simulink model "LATC_Test_Calc"  (R2021b)
settings: Solver=FixedStepDiscrete  StartTime=3849.7586  StopTime=3889.7825  FixedStep=0.01  RelTol=1e-3
values from neighbouring files (symbols this model uses):
  P_Global_CharSpd_ms : value not decoded    [PubParsGlobal.sldd]
  P_Global_SteeringAngleRatio : value not decoded    [PubParsGlobal.sldd]
  P_Global_WheelBase_m : value not decoded    [PubParsGlobal.sldd]
  P_LCS_CycleTime = 0.4 0.4 0.4 0.4 0.4 0.4 0.4 0.4 0.4 0.6 0.6 0.6 0.6 0.6 0.6 0.6 0.4 0.4 0.4 0.4 0.4 0.4 0.4 0.4 0.4 0.6 0.6 0.6 0.6 0.6 0.6 0.6 0.4 0.4 0.4 0.4 0.4 0.4 0.4 0.4 0.4 0.6 0.6 0.6 0.6 0.6 0.6 0.6 0.4 0.4 0.4 0.4 0.4 0.4 0.4 0.4 0.4 0.6 0.6 0.6 0.6 0.6 0.6 0.6 0.4 0.4 0.4 0.4 0.4 0.4 0.4 0.4 0.4 0.6 0.6 0.6 0.6 0.6 0.6 0.6 0.4 0.4 0.4 0.4 0.4 0.4 0.4 0.4 0.4 0.6 0.6 0.6 0.6 0.6 0.6 0.6 0.4 0.4 0.4 0.4    [LATC.sldd]
  P_LCS_ESS_AngleSlope_Limit = 2.9    [LATC.sldd]    (also in LCS_v05.sldd)
  P_LCS_LATC_CurOffsetVehicleSpdLimitValue_degs = 7.0    [LATC.sldd]
  P_LCS_LATC_ELKAngleSlope_ratio : value not decoded    [LATC.sldd]
  P_LCS_LATC_ELKMaxLatAcc_ms2 : value not decoded    [LATC.sldd]
  P_LCS_LATC_ESSAngleSlope_ratio : value not decoded    [LATC.sldd]
  P_LCS_LATC_ESSMaxLatAcc_ms2 : value not decoded    [LATC.sldd]
  P_LCS_LATC_LCAngleSlope_ratio : value not decoded    [LATC.sldd]
  P_LCS_LATC_LCCancleMaxLatAcc_ms2 : value not decoded    [LATC.sldd]
  P_LCS_LATC_LCEcoAngleSlope_ratio : value not decoded    [LATC.sldd]
  P_LCS_LATC_LCEcoMaxLatAcc_ms2 : value not decoded    [LATC.sldd]
  P_LCS_LATC_LCKAngleSlope_ratio : value not decoded    [LATC.sldd]
  P_LCS_LATC_LCKIEAngleSlope_ratio : value not decoded    [LATC.sldd]
  P_LCS_LATC_LCKIEMaxLatAcc_ms2 : value not decoded    [LATC.sldd]
  P_LCS_LATC_LCKMaxLatAcc_ms2 : value not decoded    [LATC.sldd]
  P_LCS_LATC_LCNormalAngleSlope_ratio : value not decoded    [LATC.sldd]
  P_LCS_LATC_LCNormalMaxLatAcc_ms2 : value not decoded    [LATC.sldd]
  P_LCS_LATC_LCSportAngleSlope_ratio : value not decoded    [LATC.sldd]
  P_LCS_LATC_LCSportMaxLatAcc_ms2 : value not decoded    [LATC.sldd]
  P_LCS_LATC_LKAAngleSlope_ratio : value not decoded    [LATC.sldd]
  P_LCS_LATC_LKAMaxLatAcc_ms2 : value not decoded    [LATC.sldd]
  P_LCS_LATC_MatrixQ1_st = 0.8 0.8 1.2 1.4 1.4 1.4 2.0 2.2 2.2 2.2 2.2 2.2 2.2 2.2 2.2 2.2 0.8 0.8 1.2 1.4 1.4 1.4 2.0 2.2 2.2 2.2 2.2 2.2 2.2 2.2 2.2 2.2 0.8 0.8 1.2 1.4 1.4 1.4 2.0 2.2 2.2 2.2 2.2 2.2 2.2 2.2 2.2 2.2 0.8 0.8 1.2 1.4 1.4 1.4 2.0 2.2 2.2 2.2 2.2 2.2 2.2 2.2 2.2 2.2 0.8 0.8 1.2 1.4 1.4 1.4 2.0 2.2 2.2 2.2 2.2 2.2 2.2 2.2 2.2 2.2 0.8 0.8 1.2 1.4 1.4 1.4 2.0 2.2 2.2 2.2 2.2 2.2 2.2 2.2 2.2 2.2 0.8 0.8 1.2 1.4    [LATC.sldd]
  P_LCS_LATC_MatrixQ3_st = 20.0 20.0 20.0 20.0 20.0 15.0 15.0 15.0 15.0 15.0 15.0 15.0 15.0 13.0 13.0 13.0 20.0 20.0 20.0 20.0 20.0 15.0 15.0 15.0 15.0 15.0 15.0 15.0 15.0 13.0 13.0 13.0 20.0 20.0 20.0 20.0 20.0 15.0 15.0 15.0 15.0 15.0 15.0 15.0 15.0 13.0 13.0 13.0 20.0 20.0 20.0 20.0 20.0 15.0 15.0 15.0 15.0 15.0 15.0 15.0 15.0 13.0 13.0 13.0 20.0 20.0 20.0 20.0 20.0 15.0 15.0 15.0 15.0 15.0 15.0 15.0 15.0 13.0 13.0 13.0    [LATC.sldd]
  P_LCS_LATC_MatrixR_st = 10.0 10.0 10.0 10.0 10.0 10.0 10.0 15.0 15.0 15.0 15.0 15.0 15.0 15.0 15.0 15.0 10.0 10.0 10.0 10.0 10.0 10.0 10.0 15.0 15.0 15.0 15.0 15.0 15.0 15.0 15.0 15.0 10.0 10.0 10.0 10.0 10.0 10.0 10.0 15.0 15.0 15.0 15.0 15.0 15.0 15.0 15.0 15.0 10.0 10.0 10.0 10.0 10.0 10.0 10.0 15.0 15.0 15.0 15.0 15.0 15.0 15.0 15.0 15.0 10.0 10.0 10.0 10.0 10.0 10.0 10.0 15.0 15.0 15.0 15.0 15.0 15.0 15.0 15.0 15.0    [LATC.sldd]
  P_LCS_LATC_StateActivAngleSlopeLimit_ratio : value not decoded    [LATC.sldd]
  P_LCS_LATC_StateActiveFlg_TabX_st : value not decoded    [LATC.sldd]
  P_LCS_LATC_StateActiveHoldTime_TabY_st : value not decoded    [LATC.sldd]
  P_LCS_LATC_StateHoldTime_st = 250.0    [LATC.sldd]
  P_LCS_LATC_TarAngleFliterWindowSize = 5.0    [LATC.sldd]
  P_LCS_LineVaildSW = 0.0    [LATC.sldd]
  P_LCS_Lookahead_Distance : value not decoded    [LATC.sldd]
  P_LCS_VehicleSpd_TabX_Kph : value not decoded    [LATC.sldd]
libraries: simulink x4
(part 3 of 4)

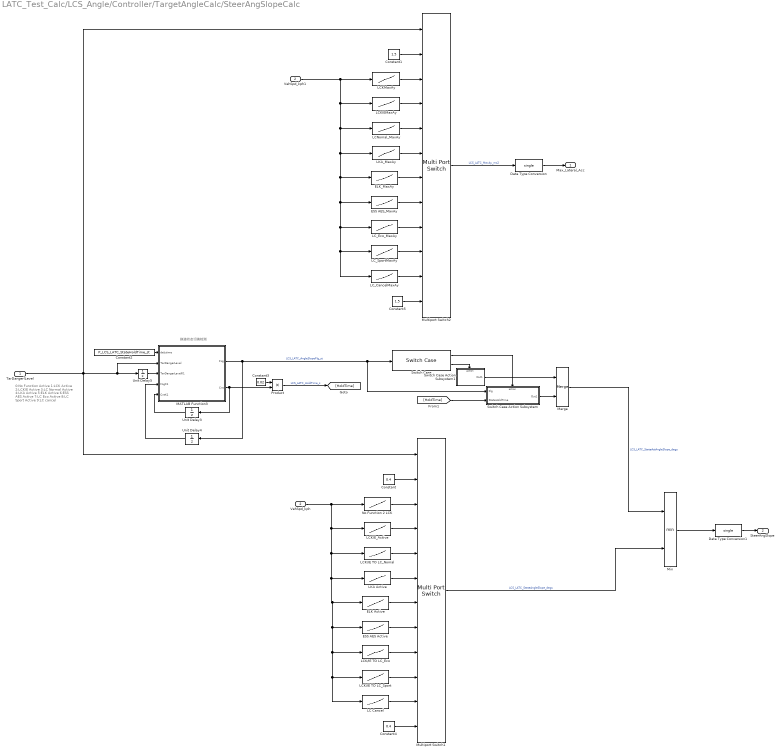
== system LATC_Test_Calc/LCS_Angle/Controller/TargetAngleCalc/SteerAngSlopeCalc ==
  note: 换道状态切换检测
  note: 0:No Function Active
      | 1:LCK Active
      | 2:LCKIE Active
      | 3:LC Normal Active
      | 4:LKA Active
      | 5:ELK Active
      | 6:ESS AES Active
      | 7:LC Eco Active
      | 8:LC Sport Active
      | 9:LC cancel
  TarDangerlLevel : Inport
  VehSpd_kph : Inport  Port=2
  Constant : Constant  Value=0.4  OutDataTypeStr=single
  Constant1 : Constant  Value=1.5  OutDataTypeStr=single
  Constant2 : Constant  Value=P_LCS_LATC_StateHoldTime_st  OutDataTypeStr=uint16
  Constant3 : Constant  Value=0.02
  Constant4 : Constant  Value=0.4  OutDataTypeStr=single
  Constant5 : Constant  Value=1.5  OutDataTypeStr=single
  Data Type Conversion : DataTypeConversion  OutDataTypeStr=single
  Data Type Conversion1 : DataTypeConversion  OutDataTypeStr=single
  ELK Active : Lookup_n-D  NumberOfTableDimensions=1  BreakpointsForDimension1=P_LCS_VehicleSpd_TabX_Kph  Table=P_LCS_LATC_ELKAngleSlope_ratio  ExtrapMethod=Clip  InternalRulePriority=Speed  RndMeth=Simplest  InputSameDT=on
  ELK_MaxAy : Lookup_n-D  NumberOfTableDimensions=1  BreakpointsForDimension1=P_LCS_VehicleSpd_TabX_Kph  Table=P_LCS_LATC_ELKMaxLatAcc_ms2  ExtrapMethod=Clip  InternalRulePriority=Speed  RndMeth=Simplest  InputSameDT=on
  ESS AES Active : Lookup_n-D  NumberOfTableDimensions=1  BreakpointsForDimension1=P_LCS_VehicleSpd_TabX_Kph  Table=P_LCS_LATC_ESSAngleSlope_ratio  ExtrapMethod=Clip  InternalRulePriority=Speed  RndMeth=Simplest  InputSameDT=on
  ESS AES_MaxAy : Lookup_n-D  NumberOfTableDimensions=1  BreakpointsForDimension1=P_LCS_VehicleSpd_TabX_Kph  Table=P_LCS_LATC_ESSMaxLatAcc_ms2  ExtrapMethod=Clip  InternalRulePriority=Speed  RndMeth=Simplest  InputSameDT=on
  LC Cancel : Lookup_n-D  NumberOfTableDimensions=1  BreakpointsForDimension1=P_LCS_VehicleSpd_TabX_Kph  Table=P_LCS_LATC_LCAngleSlope_ratio  ExtrapMethod=Clip  InternalRulePriority=Speed  RndMeth=Simplest  InputSameDT=on
  LCK/IE TO LC_Eco : Lookup_n-D  NumberOfTableDimensions=1  BreakpointsForDimension1=P_LCS_VehicleSpd_TabX_Kph  Table=P_LCS_LATC_LCEcoAngleSlope_ratio  ExtrapMethod=Clip  InternalRulePriority=Speed  RndMeth=Simplest  InputSameDT=on
  LCK/IE TO LC_Nomal : Lookup_n-D  NumberOfTableDimensions=1  BreakpointsForDimension1=P_LCS_VehicleSpd_TabX_Kph  Table=P_LCS_LATC_LCNormalAngleSlope_ratio  ExtrapMethod=Clip  InternalRulePriority=Speed  RndMeth=Simplest  InputSameDT=on
  LCK/IE TO LC_Sport : Lookup_n-D  NumberOfTableDimensions=1  BreakpointsForDimension1=P_LCS_VehicleSpd_TabX_Kph  Table=P_LCS_LATC_LCSportAngleSlope_ratio  ExtrapMethod=Clip  InternalRulePriority=Speed  RndMeth=Simplest  InputSameDT=on
  LCKIEMaxAy : Lookup_n-D  NumberOfTableDimensions=1  BreakpointsForDimension1=P_LCS_VehicleSpd_TabX_Kph  Table=P_LCS_LATC_LCKIEMaxLatAcc_ms2  ExtrapMethod=Clip  InternalRulePriority=Speed  RndMeth=Simplest  InputSameDT=on
  LCKIE_Active : Lookup_n-D  NumberOfTableDimensions=1  BreakpointsForDimension1=P_LCS_VehicleSpd_TabX_Kph  Table=P_LCS_LATC_LCKIEAngleSlope_ratio  ExtrapMethod=Clip  InternalRulePriority=Speed  RndMeth=Simplest  InputSameDT=on
  LCKMaxAy : Lookup_n-D  NumberOfTableDimensions=1  BreakpointsForDimension1=P_LCS_VehicleSpd_TabX_Kph  Table=P_LCS_LATC_LCKMaxLatAcc_ms2  ExtrapMethod=Clip  InternalRulePriority=Speed  RndMeth=Simplest  InputSameDT=on
  LCNomal_MaxAy : Lookup_n-D  NumberOfTableDimensions=1  BreakpointsForDimension1=P_LCS_VehicleSpd_TabX_Kph  Table=P_LCS_LATC_LCNormalMaxLatAcc_ms2  ExtrapMethod=Clip  InternalRulePriority=Speed  RndMeth=Simplest  InputSameDT=on
  LC_CancelMaxAy : Lookup_n-D  NumberOfTableDimensions=1  BreakpointsForDimension1=P_LCS_VehicleSpd_TabX_Kph  Table=P_LCS_LATC_LCCancleMaxLatAcc_ms2  ExtrapMethod=Clip  InternalRulePriority=Speed  RndMeth=Simplest  InputSameDT=on
  LC_Eco_MaxAy : Lookup_n-D  NumberOfTableDimensions=1  BreakpointsForDimension1=P_LCS_VehicleSpd_TabX_Kph  Table=P_LCS_LATC_LCEcoMaxLatAcc_ms2  ExtrapMethod=Clip  InternalRulePriority=Speed  RndMeth=Simplest  InputSameDT=on
  LC_SportMaxAy : Lookup_n-D  NumberOfTableDimensions=1  BreakpointsForDimension1=P_LCS_VehicleSpd_TabX_Kph  Table=P_LCS_LATC_LCSportMaxLatAcc_ms2  ExtrapMethod=Clip  InternalRulePriority=Speed  RndMeth=Simplest  InputSameDT=on
  LKA Active : Lookup_n-D  NumberOfTableDimensions=1  BreakpointsForDimension1=P_LCS_VehicleSpd_TabX_Kph  Table=P_LCS_LATC_LKAAngleSlope_ratio  ExtrapMethod=Clip  InternalRulePriority=Speed  RndMeth=Simplest  InputSameDT=on
  LKA_MaxAy : Lookup_n-D  NumberOfTableDimensions=1  BreakpointsForDimension1=P_LCS_VehicleSpd_TabX_Kph  Table=P_LCS_LATC_LKAMaxLatAcc_ms2  ExtrapMethod=Clip  InternalRulePriority=Speed  RndMeth=Simplest  InputSameDT=on
  MATLAB Function3 : MATLAB Function  TreatAsAtomicUnit=on
  Merge : Merge
  Min : MinMax  Inputs=2
  Multiport Switch1 : MultiPortSwitch  DataPortOrder=Zero-based contiguous  Inputs=11  zeroidx=on
  Multiport Switch2 : MultiPortSwitch  DataPortOrder=Zero-based contiguous  Inputs=11  zeroidx=on
  No Function 2 LCK : Lookup_n-D  NumberOfTableDimensions=1  BreakpointsForDimension1=P_LCS_VehicleSpd_TabX_Kph  Table=P_LCS_LATC_LCKAngleSlope_ratio  ExtrapMethod=Clip  InternalRulePriority=Speed  RndMeth=Simplest  InputSameDT=on
  Product : Product
  Switch Case : SwitchCase  CaseConditions={[1,2,3,4,5]}
  Switch Case Action Subsystem : Subsystem  TreatAsAtomicUnit=on
  Switch Case Action Subsystem1 : Subsystem  TreatAsAtomicUnit=on
  Unit Delay3 : UnitDelay  SampleTime=-1  HasFrameUpgradeWarning=on
  Unit Delay4 : UnitDelay  SampleTime=-1  HasFrameUpgradeWarning=on
  Unit Delay5 : UnitDelay  SampleTime=-1  HasFrameUpgradeWarning=on
  VehSpd_kph1 : InportShadow  Port=2
  Max_Lateral_Acc : Outport  OutDataTypeStr=single
  SteerAngSlope : Outport  Port=2  OutDataTypeStr=single
  wires:
  Data Type Conversion1/1 -> SteerAngSlope/1
  Data Type Conversion/1 -> Max_Lateral_Acc/1
  LCNomal_MaxAy/1 -> Multiport Switch2/5
  LKA_MaxAy/1 -> Multiport Switch2/6
  LCKMaxAy/1 -> Multiport Switch2/3
  LCKIEMaxAy/1 -> Multiport Switch2/4
  ELK_MaxAy/1 -> Multiport Switch2/7
  VehSpd_kph1/1 -> LCKMaxAy/1, LCNomal_MaxAy/1, LC_CancelMaxAy/1, LC_SportMaxAy/1, LC_Eco_MaxAy/1, ESS AES_MaxAy/1, ELK_MaxAy/1, LKA_MaxAy/1, LCKIEMaxAy/1
  ESS AES_MaxAy/1 -> Multiport Switch2/8
  LC_Eco_MaxAy/1 -> Multiport Switch2/9
  LC_SportMaxAy/1 -> Multiport Switch2/10
  LC_CancelMaxAy/1 -> Multiport Switch2/11
  Constant5/1 -> Multiport Switch2/12
  Constant1/1 -> Multiport Switch2/2
  Multiport Switch2/1 -> Data Type Conversion/1  "LCS_LATC_MaxAy_ms2"
  LC Cancel/1 -> Multiport Switch1/11
  LCK/IE TO LC_Sport/1 -> Multiport Switch1/10
  LCK/IE TO LC_Eco/1 -> Multiport Switch1/9
  ESS AES Active/1 -> Multiport Switch1/8
  Unit Delay5/1 -> MATLAB Function3/3(TarDangerLevelK1)
  VehSpd_kph/1 -> LCKIE_Active/1, LKA Active/1, ELK Active/1, ESS AES Active/1, LCK/IE TO LC_Eco/1, LCK/IE TO LC_Sport/1, LC Cancel/1, LCK/IE TO LC_Nomal/1, No Function 2 LCK/1
  ELK Active/1 -> Multiport Switch1/7
  LCKIE_Active/1 -> Multiport Switch1/4
  Unit Delay3/1 -> MATLAB Function3/5(CntK1)
  Unit Delay4/1 -> MATLAB Function3/4(FLgK1)
  Constant/1 -> Multiport Switch1/2
  MATLAB Function3/2(Cnt) -> Product/2, Unit Delay3/1
  MATLAB Function3/1(FLg) -> Switch Case/1, Switch Case Action Subsystem/1(Flg), Unit Delay4/1  "LCS_LATC_AngleSlopeFlg_st"
  Constant2/1 -> MATLAB Function3/1(delytime)
  Multiport Switch1/1 -> Min/2  "LCS_LATC_StateAngleSlope_degs"
  No Function 2 LCK/1 -> Multiport Switch1/3
  LKA Active/1 -> Multiport Switch1/6
  Constant4/1 -> Multiport Switch1/12
  Constant3/1 -> Product/1
  Product/1 -> [HoldTime]  "LCS_LATC_HoldTime_s"
  Min/1 -> Data Type Conversion1/1
  LCK/IE TO LC_Nomal/1 -> Multiport Switch1/5
  Switch Case/1 -> Switch Case Action Subsystem/Action
  Switch Case/2 -> Switch Case Action Subsystem1/Action
  [HoldTime] -> Switch Case Action Subsystem/2(StateHoldTime)
  Switch Case Action Subsystem/1(Out1) -> Merge/2
  Switch Case Action Subsystem1/1(Out1) -> Merge/1
  Merge/1 -> Min/1  "LCS_LATC_StateActAngleSlope_degs"
  TarDangerlLevel/1 -> MATLAB Function3/2(TarDangerLevel), Unit Delay5/1, Multiport Switch2/1, Multiport Switch1/1

== system LATC_Test_Calc/LCS_Angle/Controller/Understeer&Offset_Calc/Enabled Subsystem ==
  AckConst : Inport
  Raw : Inport  Port=2
  Enable : EnablePort
  Constant1 : Constant  Value=2  OutDataTypeStr=single
  Constant2 : Constant  Value=0.02  OutDataTypeStr=single
  Constant7 : Constant  Value=P_Global_SteeringAngleRatio
  Constant8 : Constant  Value=57.3  OutDataTypeStr=single
  FilterTime2 : Product  Inputs=4  RndMeth=Zero
  Product2 : Product  Inputs=*/  RndMeth=Zero
  Product6 : Product  RndMeth=Zero
  Sum6 : Sum  Inputs=+-
  Sum7 : Sum
  Unit Delay : UnitDelay  SampleTime=-1  HasFrameUpgradeWarning=on
  SteerAngleOffset_deg : Outport
  wires:
  Sum7/1 -> SteerAngleOffset_deg/1, Unit Delay/1
  Unit Delay/1 -> Sum6/2, Sum7/2
  Constant2/1 -> Product2/1
  Sum6/1 -> Product6/2
  Product2/1 -> Product6/1
  Product6/1 -> Sum7/1
  Constant7/1 -> FilterTime2/1
  Constant8/1 -> FilterTime2/2
  AckConst/1 -> FilterTime2/3
  Raw/1 -> FilterTime2/4
  FilterTime2/1 -> Sum6/1
  Constant1/1 -> Product2/2

== system LATC_Test_Calc/LCS_Angle/Controller/TargetAngleCalc/SteerAngSlopeCalc/Switch Case Action Subsystem ==
  Flg : Inport
  StateHoldTime : Inport  Port=2
  Action Port : ActionPort  ActionPortLabel=case [ 1 2 3 4 5 ]:
  LC_start_slope : Lookup_n-D  BreakpointsForDimension1=P_LCS_LATC_StateActiveFlg_TabX_st  BreakpointsForDimension2=P_LCS_LATC_StateActiveHoldTime_TabY_st  Table=P_LCS_LATC_StateActivAngleSlopeLimit_ratio  ExtrapMethod=Clip  UseLastTableValue=on  InternalRulePriority=Speed  OutDataTypeStr=single  RndMeth=Simplest
      settings: InputPortMap=u0,u1
  Out1 : Outport
  wires:
  Flg/1 -> LC_start_slope/1
  LC_start_slope/1 -> Out1/1
  StateHoldTime/1 -> LC_start_slope/2

== system LATC_Test_Calc/LCS_Angle/Controller/TargetAngleCalc/SteerAngSlopeCalc/Switch Case Action Subsystem1 ==
  Action Port : ActionPort  ActionPortLabel=default:
  Constant : Constant  Value=100  OutDataTypeStr=single
  Out1 : Outport
  wires:
  Constant/1 -> Out1/1

== matlab function LATC_Test_Calc/LCS_Angle/Trajectory_Planning/QP_Path/path planning with quadratic programming (qp) ==
  data: qp_path_s output; l_min input; qp_path_l output; l_max input; w_cost_l input; w_cost_dl input; w_cost_ddl input; w_cost_dddl input; w_cost_centre input; w_cost_end_l input; w_cost_end_dl input; w_cost_end_ddl input; host_d1 input; host_d2 input; host_w input; plan_start_s input; plan_start_l input; plan_start_dl input; plan_start_ddl input; qp_path_dl output; qp_path_ddl output; delta_dl_max input; delta_ddl_max input; dp_path_l_final input
function [qp_path_s,qp_path_l,qp_path_dl,qp_path_ddl] = ...
fcn(l_min,l_max,w_cost_l,w_cost_dl,w_cost_ddl,w_cost_dddl,w_cost_centre,w_cost_end_l,w_cost_end_dl,w_cost_end_ddl,...
    host_d1,host_d2,host_w,...
    plan_start_s,plan_start_l,plan_start_dl,plan_start_ddl,delta_dl_max,delta_ddl_max,dp_path_l_final)
% 路径二次规划
% 0.5*x'Hx + f'*x = min
% subject to A*x <= b
%            Aeq*x = beq
%            lb <= x <= ub;
% 输入：l_min l_max 点的凸空间
%       w_cost_l 参考线代价
%       w_cost_dl ddl dddl 光滑性代价
%       w_cost_centre 凸空间中央代价
%       w_cost_end_l dl dd1 终点的状态代价 (希望path的终点状态为(0,0,0))
%       host_d1,d2 host质心到前后轴的距离
%       host_w host的宽度
%       plan_start_l,dl,ddl 规划起点
% 输出 qp_path_l dl ddl 二次规划输出的曲线
% coder.extrinsic("quadprog");
% 待优化的变量的数量
n = single(20);
%输出初始化
qp_path_l = single(zeros(n,1));
qp_path_dl = single(zeros(n,1));
qp_path_ddl = single(zeros(n,1));
qp_path_s = single(zeros(n,1));
% 构建约束
% subject to A*x <= b
%            Aeq*x = beq
%            lb <= x <= ub;
% Aeq_sub = [1 ds ds^2/3 -1 0 ds^2/6;
%            0 1  ds/2   0 -1 ds/2];
% x = [Li Li' Li'' Li+1 Li+1' Li+1'']
% beq = [0;0]

% 两点间距
ds = single(3);
% 60个点隔2个取一个
for i = 1:n
    qp_path_s(i) = plan_start_s + (i-1)*ds;
end

%-------------------以下为约束生成----------------
% 等式约束
Aeq = single(zeros(2*n-2,3*n));
beq = single(zeros(2*n-2,1));
% 两点间距
Aeq_sub = single([1 ds ds^2/3 -1 0 ds^2/6;
                  0 1  ds/2   0 -1 ds/2]);
% 通过Aeq_sub填充Aeq ,beq不变全为0
for i = 1:n-1
    row = 2*i-1;
    col = 3*i-2;  
    Aeq(row:row+1,col:col+5) = Aeq_sub;  
end
% 不等式约束 A*x <= b
% 车辆四个角点在凸空间内
% 不等式矩阵初始化
A = single(zeros(8*n, 3*n));
b = single(zeros(8*n, 1));
%构建A_sub
d1 = host_d1;%质心到前保险杠距离
d2 = host_d2;%质心到后保险杠距离
w = host_w;%车宽
A_sub = [1  d1 0;
         1  d1 0;
         1 -d2 0;
         1 -d2 0;
        -1 -d1 0;
        -1 -d1 0;
        -1  d2 0;
        -1  d2 0];
% 生成A矩阵
for i=1:n
    row = 8*i-7;
    col = 3*i-2;
    A(row:row+7,col:col+2) = A_sub;
end
% 这里没有对曲率做强制约束，并不好
% 可以用 |dl(i+1) - dl(i)|/ds <= kappa_max 近似去约束曲率
% 以下为对曲率进行约束
% A_cur = single(zeros(n-1,3*n));
% b_cur = single(ones(n-1,1)*kappa_max);
% A_cur_sub = single([-1/ds 0 0 1/ds 0 0]);
% for i = 1:n-1
%     row = i;
%     col = 3*i-2;
%     A_cur(row,col:col+5) = A_cur_sub;
% end
% A_Cur = [A_cur;
%         -1*A_cur;];
% B_Cur = [b_cur;
%          b_cur;];

% 更新：加入 dl(i+1) - dl(i) ddl(i+1) - ddl(i) 的约束
A_dl_minus = zeros(n - 1,3*n);
b_dl_minus = zeros(n - 1,1);
A_ddl_minus = zeros(n - 1,3*n);
b_ddl_minus = zeros(n - 1,1);
for i = 1:n-1
    row = i;
    col = 3*i - 2;
    A_dl_minus(row,col:col+5) = [0 -1 0 0 1 0];
    b_dl_minus(row) = delta_dl_max;
    A_ddl_minus(row,col:col+5) = [0 0 -1 0 0 1];
    b_ddl_minus(row) = delta_ddl_max;
end
% -max < a*x < max => ax < max && -ax < -(-max)
A_minus = [A_dl_minus;
          -A_dl_minus;
           A_ddl_minus;
          -A_ddl_minus];
b_minus = [b_dl_minus;
           b_dl_minus;
          b_ddl_minus;
          b_ddl_minus]; 



% 生成b矩阵
% 只要找到四个角点所对应的l_min l_max 即可
% 。。。。。。。。。。。。。。
%    [    .   ]<- 
%    [        ]
% 。。。。。。。。。。。。。
front_index = ceil(d1/ds);
back_index = ceil(d2/ds);

for i=2:n
%     index1 = min(i+front_index,n);
%     index2 = max(i-back_index,1);
    index1 = min(3*i - 2 + front_index,n);
    index2 = max(3*i - 2 - back_index,1);
    b(8*i - 7:8*i,1) = [l_max(index1) - w/2;
                        l_max(index1) + w/2;
                        l_max(index2) - w/2;
                        l_max(index2) + w/2;
                       -l_min(index1) + w/2;
                       -l_min(index1) - w/2;
                       -l_min(index2) + w/2;
                       -l_min(index2) - w/2;];
end
%生成边界约束lb ub。主要是对规划起点做约束
lb = single(ones(3*n,1)*-inf);
ub = single(ones(3*n,1)*inf);
lb(1) = plan_start_l;
lb(2) = plan_start_dl;
lb(3) = plan_start_ddl;
ub(1) = lb(1);
ub(2) = lb(2);
ub(3) = lb(3);
% for i = 2:n
%     lb(3*i - 1) = -2; %约束 l'
%     ub(3*i - 1) = 2;
%     lb(3*i) = -0.1; %约束 l''
%     ub(3*i) = 0.1;
% end
%------------------以上约束生成完毕--------------------------
%------------------生成H矩阵--------------------------------
% 矩阵初始化
H_L = zeros(3*n, 3*n);
H_DL = zeros(3*n, 3*n);
H_DDL = zeros(3*n, 3*n);
H_DDDL = zeros(n-1, 3*n);
% H_CENTRE = zeros(3*n, 3*n);
H_L_END = zeros(3*n, 3*n);
H_DL_END = zeros(3*n, 3*n);
H_DDL_END = zeros(3*n, 3*n);
% 生成H_L,H_DL,H_DDL,H_CENTRE
for i = 1:n
    H_L(3*i - 2,3*i - 2) = 1;
    H_DL(3*i - 1,3*i - 1) = 1;
    H_DDL(3*i, 3*i) = 1;
end
H_CENTRE = H_L; %尽量沿着目标线走
% 生成H_DDDL;
H_dddl_sub = [0 0 1 0 0 -1];
for i = 1:n-1
    row = i;
    col = 3*i - 2;
    H_DDDL(row,col:col + 5) = H_dddl_sub;
end
% 生成H_L_END H_DL_END H_DDL_END
H_L_END(3*n - 2,3*n - 2) = 1;
H_DL_END(3*n - 1,3*n - 1) = 1;
H_DDL_END(3*n,3*n) = 1;
% 生成二次规划的H
% 生成二次规划的H 因为ds ！= 1 所以 dddl = delta_ddl/ds;
H = w_cost_l * (H_L'*H_L) + w_cost_dl * (H_DL'*H_DL) + w_cost_ddl * (H_DDL'*H_DDL)...
   +w_cost_dddl * (H_DDDL'*H_DDDL)/ds + w_cost_centre * (H_CENTRE'*H_CENTRE) + w_cost_end_l * (H_L_END'*H_L_END)...
   +w_cost_end_dl * (H_DL_END'* H_DL_END) + w_cost_ddl * (H_DDL_END'*H_DDL_END);
H = single(2 * H);
%---------------------------生成H完毕------------------------------
% 0.5*x'Hx + f'*x = min
% 生成f
f = single(zeros(3*n,1));
% centre_line = 0.5 * (l_min + l_max);
centre_line = 0.5 * (l_min + l_max); % 此时centre line 还是60个点
for i = 1:n
    f(3*i - 2) = -2 * centre_line(3*i - 2);
end
% 避免centreline权重过大影响轨迹平顺性
for i = 1:n
    if abs(f(i)) > 0.6
        f(i) = w_cost_centre * f(i);
    end
end

% centre_line = dp_path_l_final;
% for i = 1:n
%     f(3*i - 2) = -2 * centre_line(3*i - 2);
% end
% f = w_cost_centre * f;

% 终点要接近end_l dl ddl desire
%  期望的终点状态
end_l_desire = 0;
end_dl_desire = 0;
end_ddl_desire = 0;
f(3*n - 2) = f(3*n - 2) -2 * end_l_desire * w_cost_end_l;
f(3*n - 1) = f(3*n - 1) -2 * end_dl_desire * w_cost_end_dl;
f(3*n) = f(3*n) -2 * end_ddl_desire * w_cost_end_ddl;
%-----------f构造完毕---------------------------------------------
% 0.5*x'Hx + f'*x = min
% subject to A*x <= b
%            Aeq*x = beq
%            lb <= x <= ub;

% X = quadprog(H,f,A,b,Aeq,beq,lb,ub);

%---------改造求解---------------
% J = 0.5x'Hx + f'x = min
% A_Const * x <= b
A_Const = single([A;eye(3*n,3*n);-1*eye(3*n,3*n);Aeq;-1*Aeq;A_minus]);
b_Const = single([b;ub;-1*lb;beq;-1*beq;b_minus]);

X = MPC_Solver_QPhild(H,f,A_Const,b_Const);

for i = 1:n
    qp_path_l(i) = X(3*i - 2);
    qp_path_dl(i) = X(3*i - 1);
    qp_path_ddl(i) = X(3*i);
end

end
function eta = MPC_Solver_QPhild(H,f,A_Const,b)
% 二次规划
% 该算法是原始对偶算法，该方法充分的剖析了优化问题的结构，是求解二次规划问题的一个较好的算法。
% J = 0.5x'Hx + f'x = min
% A_Const*x <= b
[n1,~] = size(A_Const);
eta = -H\f;
kk = uint8(0);
for i = 1:n1
    if(A_Const(i,:)*eta>b(i))
        kk = kk+uint8(1);
    else
        kk = kk+uint8(0);
    end
end
if kk == uint8(0)
    return;
end
P = A_Const*(H\A_Const');
d = (A_Const*(H\f)+b);
[n,m] = size(d);
x_ini = zeros(n,m);
lambda = x_ini;
al = single(10);
for km = 1:38
    lambda_p = lambda;
    for i = 1:n
        w = P(i,:)*lambda - P(i,i)*lambda(i,1);
        w = w + d(i,1);
        la = -w/P(i,i);
        lambda(i,1) = max(0,la);
    end
    al = (lambda - lambda_p)'*(lambda - lambda_p);
    if(al<10e-8)
        break
    end
end
eta = -H\f -H\A_Const'*lambda;
end

== matlab function LATC_Test_Calc/LCS_Angle/Trajectory_Planning/MATLAB Function14 ==
  data: X input; y output; Y input
function y = fcn(X,Y)

y = zeros(length(X),9);
for i = 1:1:length(X)
    y(i,1) = X(i);
    y(i,2) = Y(i);
    y(i,3) = 0;
    y(i,4) = 0;
    y(i,5) = 1;
    y(i,6) = i;
    y(i,7) = 0;
    y(i,8) = 1;
end
end

== matlab function LATC_Test_Calc/LCS_Angle/Controller/StateErrorCalc/MATLAB Function ==
  data: Lookahead_Distance input; Ego_X input; Ego_Y input; Traj_X input; Traj_Y input; Traj_Heading input; Traj_Kappa input; Traj_S input; lookahead_Pt_X output; Target_Pt_X input; Target_Pt_Y input; Target_Pt_S input; lookahead_Pt_Y output; lookahead_Pt_Heading output; lookahead_Pt_Kappa output single; Lookahead_Pt_Num output
%% 为横向控制找预瞄点
function [lookahead_Pt_X,lookahead_Pt_Y,lookahead_Pt_Heading,lookahead_Pt_Kappa,Lookahead_Pt_Num]= ...
QueryLookaheadPointByPosition(Lookahead_Distance,Ego_X,Ego_Y,Traj_X,Traj_Y,Traj_Heading,Traj_Kappa,Traj_S,Target_Pt_X,Target_Pt_Y,Target_Pt_S)

    target_dist=((Target_Pt_X-Ego_X)^2+((Target_Pt_Y-Ego_Y)^2))^0.5;
    lookahead_index=0;
    lookahead_dist=target_dist;
    for i=1:length(Traj_X)
        %找到轨迹上累积弧长之差超过此距离的点作为预瞄点 
        %到目标点距离，再加上第i个点与目标点的弧长s之差刚好大于预瞄距离的那个点
        lookahead_dist=lookahead_dist+Traj_S(i,1)-Target_Pt_S(1,1);
        
        if(lookahead_dist>=Lookahead_Distance)
            lookahead_index = i;
            lookahead_Pt_X= Traj_X(lookahead_index,1);
            lookahead_Pt_Y= Traj_Y(lookahead_index,1);
            lookahead_Pt_Heading= Traj_Heading(lookahead_index,1);
            lookahead_Pt_Kappa= Traj_Kappa(lookahead_index,1);
            Lookahead_Pt_Num = i;
            return
        end
        %若遍历到最后一个点也没有大于lookahead_station的就取最后一个点
        lookahead_Pt_X= Traj_X(i,1);
        lookahead_Pt_Y= Traj_Y(i,1);
        lookahead_Pt_Heading= Traj_Heading(i,1);
        lookahead_Pt_Kappa= Traj_Kappa(i,1);
    end
    Lookahead_Pt_Num = i;
end

== matlab function LATC_Test_Calc/LCS_Angle/Controller/StateErrorCalc/MATLAB Function2 ==
  data: Ego_X input; Ego_Y input; Ego_Heading input; Ego_Spd input; Ego_Acc input; Ego_YawRate input; lookahead_Pt_X input; lookahead_Pt_Y input; lookahead_Pt_Heading input; lookahead_Pt_Kappa input; Project_Pt_X input; Project_Pt_Y input; Project_Pt_Heading input; Project_Pt_Kappa input; lat_error output; lat_error_rate output; heading_error output; heading_error_rate output; lat_error_lookahead output; lat_error_rate_lookahead output; heading_error_lookahead output; heading_error_rate_lookahead output
function [lat_error,lat_error_rate,heading_error,heading_error_rate,lat_error_lookahead,lat_error_rate_lookahead,heading_error_lookahead,heading_error_rate_lookahead] ...
          = ComputeLatErrors(Ego_X,Ego_Y,Ego_Heading,Ego_Spd,Ego_Acc,Ego_YawRate,lookahead_Pt_X,lookahead_Pt_Y,lookahead_Pt_Heading,lookahead_Pt_Kappa,Project_Pt_X,Project_Pt_Y,Project_Pt_Heading,Project_Pt_Kappa)
    %% 横向控制中的误差计算  
    % 感觉存在问题，打算计算两套误差状态，一个是基于车辆与垂直点的误差，一个是车辆与预瞄点的误差。再加上前边车辆的位置推算模块
    
    % 角度误差计算
    curr_heading = Ego_Heading;
    heading_error = curr_heading-Project_Pt_Heading; % 车辆朝向角与垂直点朝向角误差
    heading_error = NormalizeAngle(heading_error);
    heading_error_lookahead = curr_heading-lookahead_Pt_Heading; % 车辆朝向角与预瞄点朝向误差
    heading_error_lookahead = NormalizeAngle(heading_error_lookahead);
    % 垂直点偏差计算
    X_curr = Ego_X;
    Y_curr = Ego_Y;
    dx = X_curr - Project_Pt_X;
    dy = Y_curr - Project_Pt_Y;
    lat_error = cos(Project_Pt_Heading)*dy-sin(Project_Pt_Heading)*dx;
    lat_error_rate=Ego_Spd*sin(heading_error);
    Project_Pt_YawRate = Project_Pt_Kappa*Ego_Acc;
    heading_error_rate = Ego_YawRate-Project_Pt_YawRate;
    % 预瞄点的偏差计算
    dx_pre = X_curr - lookahead_Pt_X;
    dy_pre = Y_curr - lookahead_Pt_Y;
    lat_error_lookahead = cos(lookahead_Pt_Heading)*dy_pre-sin(lookahead_Pt_Heading)*dx_pre;
    lat_error_rate_lookahead=Ego_Spd*sin(heading_error_lookahead);
    lookahead_Pt_YawRate = lookahead_Pt_Kappa*Ego_Acc;
    heading_error_rate_lookahead = Ego_YawRate-lookahead_Pt_YawRate;
end
function res_angle=NormalizeAngle(origin_angle)
%% 角度规范化，heading角在-pi~pi之间
    res_angle=mod(origin_angle+pi,2*pi);
    if (res_angle<0)
        res_angle=res_angle+2*pi;
    end
    res_angle=res_angle-pi;
end

% tor=[cos(thetar);sin(thetar)];
% nor=[-sin(thetar);cos(thetar)];
% d_err=[x-xr;y-yr];
% ed=nor'*d_err;
% es=tor'*d_err;
% %projection_point_thetar=thetar(dmin);%apollo
% projection_point_thetar=thetar+kappar*es;
% ed_dot=vy*cos(phi-projection_point_thetar)+vx*sin(phi-projection_point_thetar);
% %%%%%%%%%
% ephi=sin(phi-projection_point_thetar);
% %%%%%%%%%
% ss_dot=vx*cos(phi-projection_point_thetar)-vy*sin(phi-projection_point_thetar);
% s_dot=ss_dot/(1-kappar*ed);
% ephi_dot=phi_dot-kappar*s_dot;

== matlab function LATC_Test_Calc/LCS_Angle/Trajectory_Planning/MATLAB Function3 ==
  data: X input; y output; Y input
function y = fcn(X,Y)

y = zeros(length(X),9);
for i = 1:1:length(X)
    y(i,1) = X(i);
    y(i,2) = Y(i);
    y(i,3) = 0;
    y(i,4) = 0;
    y(i,5) = 1;
    y(i,6) = i;
    y(i,7) = 0;
    y(i,8) = 1;
end
end

== matlab function LATC_Test_Calc/LCS_Angle/Trajectory_Planning/DP_Path/path decision with dynamic planning(dp) ==
  data: obs_s_set input; dp_path_s output; obs_l_set input; plan_start_s input; plan_start_l input; plan_start_dl input; plan_start_dll input; w_cost_collision input; w_cost_smooth_dl input; w_cost_smooth_ddl input; w_cost_smooth_dddl input; w_cost_ref input; row input; col input; sample_s input; sample_l input; dp_path_l output
function [dp_path_s,dp_path_l] = fcn(obs_s_set,obs_l_set,plan_start_s,plan_start_l,plan_start_dl,...
    plan_start_dll,w_cost_collision,w_cost_smooth_dl,w_cost_smooth_ddl,w_cost_smooth_dddl,w_cost_ref,row,col,sample_s,sample_l)
%该函数为路径决策算法动态规划的主函数
% 输入：obs s l set 筛选后的障碍物sl信息
%       plan_start s l dl ddl 规划起点信息
%       w_cost_obs,w_cost_smooth_dl,w_cost_smooth_ddl,w_cost_smooth_dddl,w_cost_ref动态规划代价权重
%       row col 动态规划采样点的行数和列数(row必须是奇数，col必须是6)
%       sample_s,sample_l 采样的s l 长度
% 输出：dp_path_l,dp_path_s 动态规划的路径sl,此路径不包含规划起点  

%动态规划最优的数据结构是结构体矩阵，但是simulink不支持结构体矩阵，所以动态规划算法写的相对难以理解

% 用结构体矩阵进行编程
Serial_index = uint8(zeros(1,2));Node_sl = single(zeros(1,2));Node_cost = single(ones(1,1)*inf);FatherNode_index = uint8(zeros(1,2));
DP_Nodes = repmat(struct('Serial_Index',Serial_index,'Node_SL',Node_sl,'Node_Cost',Node_cost,'FatherNode_Index',FatherNode_index),50,50);
%构建结构体数组时需要明确指出大小，如果传进来，则不能运行，可能是simulink机制的问题。因此先定义50*50的作为缓冲
for i = 1:col
    for j = 1:row
        DP_Nodes(j,i).Serial_Index = uint8([j,i]);
        DP_Nodes(j,i).Node_SL = single([(plan_start_s+i*sample_s),((row + 1)/2-j)*sample_l]);
    end
end
%计算起点到第一列的cost
for i=1:row
    DP_Nodes(i,1).Node_Cost = CalcStartCost(plan_start_s,plan_start_l,plan_start_dl,...
    plan_start_dll,i,sample_s,sample_l,w_cost_collision,w_cost_smooth_dl,...
    w_cost_smooth_ddl,w_cost_smooth_dddl,w_cost_ref,obs_s_set,obs_l_set,row);
end
% 计算从第第一列到最后一列的cost
for i = 2:col
    for j = 1:row
        %计算当前node(i,j)的s l
        cur_node_s = DP_Nodes(j,i).Node_SL(1,1);
        cur_node_l = DP_Nodes(j,i).Node_SL(1,2);
        %遍历前一列的节点
        for k = 1:row
            pre_node_s = DP_Nodes(k,i-1).Node_SL(1,1);
            pre_node_l = DP_Nodes(k,i-1).Node_SL(1,2);
            cost_neighbour = CalcNeighbourCost(pre_node_s,pre_node_l,cur_node_s,cur_node_l,w_cost_collision,...
                w_cost_smooth_dl,w_cost_smooth_ddl,w_cost_smooth_dddl,w_cost_ref,obs_s_set,obs_l_set);
            %起点到上一列的cost值
            precol_min_cost = DP_Nodes(k,i-1).Node_Cost(1,1);
            cost_temp = precol_min_cost + cost_neighbour;
            if cost_temp < DP_Nodes(j,i).Node_Cost(1,1)
                DP_Nodes(j,i).Node_Cost(1,1) = cost_temp;
                %把最优路径上一列节点的行号记录下来
                DP_Nodes(j,i).FatherNode_Index = uint8([k,i-1]);
            end
        end       
    end
end
% 找出最后一列最小cost索引号
costs_temp = single(ones(50,1)*inf);
for i=1:1:row
    costs_temp(i,1) = DP_Nodes(i,col).Node_Cost;
end
% [Min_cost,Min_cost_Index] = min(costs_temp,[],1);
[~,Min_cost_Index] = min(costs_temp,[],1);
%动态规划最优路径,从后往前逆推，根据父节点往前取出每个节点的SL
dp_path_s = single(ones(15,1)*-1);
dp_path_l = single(ones(15,1)*-1);

MinCost_Index_temp = uint8(Min_cost_Index);
for i = col:-1:1
    dp_path_s(i+1) = DP_Nodes(MinCost_Index_temp,i).Node_SL(1,1);
    dp_path_l(i+1) = DP_Nodes(MinCost_Index_temp,i).Node_SL(1,2);
    MinCost_Index_temp = DP_Nodes(MinCost_Index_temp,i).FatherNode_Index(1,1);
end
% 把起点放到第一个位置
dp_path_s(1) = plan_start_s;
dp_path_l(1) = plan_start_l;
end

function cost = CalcNeighbourCost(pre_node_s,pre_node_l,cur_node_s,cur_node_l,w_cost_collision,...
    w_cost_smooth_dl,w_cost_smooth_ddl,w_cost_smooth_dddl,w_cost_ref,obs_s_set,obs_l_set)
% 该函数将计算相邻两个节点之间的cost
  
    start_l = pre_node_l;
    start_dl = single(0);
    start_ddl = single(0);
    end_l = cur_node_l;
    end_dl = single(0);
    end_ddl = single(0);
    start_s = pre_node_s;
    end_s = cur_node_s;
    coeff = CalcQuinticCoeffient(start_l,start_dl,start_ddl,end_l,end_dl,end_ddl,start_s,end_s);
    a0 = coeff(1);
    a1 = coeff(2);
    a2 = coeff(3);
    a3 = coeff(4);
    a4 = coeff(5);
    a5 = coeff(6);
    % 取10个点计算cost
    ds = single(zeros(10,1));
    l = single(zeros(10,1));
    dl = single(zeros(10,1));
    ddl = single(zeros(10,1));
    dddl = single(zeros(10,1));
    for i = 1:10
        ds(i) = start_s + (i-1)*(end_s - start_s)/10;
    end
    l = a0 * ones(10,1) + a1 * ds + a2 * ds.^2 + a3 * ds.^3 + a4 * ds.^4 + a5 * ds.^5;
    dl = a1 * ones(10,1) + 2 * a2 * ds + 3 * a3 * ds.^2 + 4 * a4 * ds.^3 + 5 * a5 * ds.^4;
    ddl = 2 * a2 * ones(10,1) + 6 * a3 * ds + 12 * a4 * ds.^2 + 20 * a5 * ds.^3;
    dddl = 6 * ones(10,1) * a3 + 24 * a4 * ds + 60 * a5 * ds.^2;
    cost_smooth = w_cost_smooth_dl * (dl' * dl) + w_cost_smooth_ddl * (ddl' * ddl) + w_cost_smooth_dddl * (dddl' * dddl);
    for i = 1:length(ddl)
        if abs(ddl(i))> 0.5 || abs(atan(dl(i))) > 0.4*pi
            cost_smooth = cost_smooth + 1e7;
            break;
        end
    end
    cost_ref = w_cost_ref * (l' * l);
    cost_collision = single(0);
    for i = 1:length(obs_s_set)
        if isnan(obs_s_set(i))
            break;
        end
        dlon = ones(10,1) * obs_s_set(i) - ds;
        dlat = ones(10,1) * obs_l_set(i) - l;
        %这里做了非常简化的质点模型，认为障碍物就是一个点
        square_d = dlon.^2 + dlat.^2;
        cost_collision_once = CalcObsCost(w_cost_collision,square_d);
        cost_collision = cost_collision + cost_collision_once;
        % 判断障碍物的左右
        v1 = [ds(end);l(end)] - [ds(1);l(1)];
        v2 = [obs_s_set(i);obs_l_set(i)] - [ds(1);l(1)];
        flag = v1(1)*v2(2) - v1(2)*v2(1);
        if flag < 0 && cost_collision > 0
            cost_collision = cost_collision - 1000;
        end
    end
    
    cost = cost_collision + cost_smooth + cost_ref;


end

function cost = CalcStartCost(begin_s,begin_l,begin_dl,begin_ddl,cur_node_row,sample_s,sample_l,w_cost_collision,...
    w_cost_smooth_dl,w_cost_smooth_ddl,w_cost_smooth_dddl,w_cost_ref,obs_s_set,obs_l_set,row)
    %该函数将计算起点到第一层的cost
    start_l = begin_l;
    start_dl = begin_dl;
    start_ddl = begin_ddl;
    %  . . .
    %  . . . row = 3 中间的行号 = (row + 1) /2 = 2
    %  . . .
    end_l = ((row + 1)/2 - cur_node_row)*sample_l;
    end_dl = 0;
    end_ddl = 0;
    start_s = begin_s;
    end_s = begin_s + sample_s;
    coeff = CalcQuinticCoeffient(start_l,start_dl,start_ddl,end_l,end_dl,end_ddl,start_s,end_s);
    a0 = coeff(1);
    a1 = coeff(2);
    a2 = coeff(3);
    a3 = coeff(4);
    a4 = coeff(5);
    a5 = coeff(6);
    % 取10个点计算cost
    ds = zeros(10,1);
    l = zeros(10,1);
    dl = zeros(10,1);
    ddl = zeros(10,1);
    dddl = zeros(10,1);
    for i = 1:10
        ds(i) = start_s + (i-1)*sample_s/10;
    end
    l = a0 * ones(10,1) + a1 * ds + a2 * ds.^2 + a3 * ds.^3 + a4 * ds.^4 + a5 * ds.^5;
    dl = a1 * ones(10,1) + 2 * a2 * ds + 3 * a3 * ds.^2 + 4 * a4 * ds.^3 + 5 * a5 * ds.^4;
    ddl = 2 * a2 * ones(10,1) + 6 * a3 * ds + 12 * a4 * ds.^2 + 20 * a5 * ds.^3;
    dddl = 6 * ones(10,1) * a3 + 24 * a4 * ds + 60 * a5 * ds.^2;
    cost_smooth = w_cost_smooth_dl * (dl' * dl) + w_cost_smooth_ddl * (ddl' * ddl) + w_cost_smooth_dddl * (dddl' * dddl);
    for i = 1:length(dl)
        if abs(ddl(i))> 0.5 || abs(atan(dl(i))) > 0.4*pi
            cost_smooth = cost_smooth + 1e7;
            break;
        end
    end
    cost_ref = w_cost_ref * (l' * l);
    cost_collision = single(0);
    for i = 1:length(obs_s_set)
        if isnan(obs_s_set(i))
            break;
        end
        dlon = ones(10,1) * obs_s_set(i) - ds;
        dlat = ones(10,1) * obs_l_set(i) - l;
        %这里做了非常简化的质点模型，认为障碍物就是一个点
        square_d = dlon.^2 + dlat.^2;
        cost_collision_once = CalcObsCost(w_cost_collision,square_d);
        cost_collision = cost_collision + cost_collision_once;
        % 判断障碍物的左右
        v1 = [ds(end);l(end)] - [ds(1);l(1)];
        v2 = [obs_s_set(i);obs_l_set(i)] - [ds(1);l(1)];
        flag = v1(1)*v2(2) - v1(2)*v2(1);
        if flag < 0 && cost_collision > 0
            cost_collision = cost_collision - 1000;
        end
    end
    
    cost = cost_collision + cost_smooth + cost_ref;
        
end

function obs_cost = CalcObsCost(w_cost_collision,square_d)
%该函数将计算障碍物的距离代价
% 暂定超过4米的cost为0 在4到3米的cost为1000/squard_d,在小于3米的cost为w_cost_collision
%   cost = 0;
%   for i = 1:length(square_d)
%       if (square_d(i) < 16 && square_d(i) > 9) 
%           cost = cost + 500/square_d(i);
%       elseif (square_d(i) <= 9)
%           cost = cost + w_cost_collision;
%       end
%   end
%   obs_cost = cost;
min_d = inf;
for i = 1:length(square_d)
    min_d = double(min(min_d,square_d(i)));
end
    obs_cost = w_cost_collision * 10^(-min_d/3);
end

function coeff = CalcQuinticCoeffient(start_l,start_dl,start_ddl,end_l,end_dl,end_ddl,start_s,end_s)
    % l = a0 + a1*s + a2*s^2 + a3*s^3 + a4*s^4 + a5*s^5
    % l' = a1 + 2 * a2 * s + 3 * a3 * s^2 + 4 * a4 * s^3 + 5 * a5 * s^4
    % l'' = 2 * a2 + 6 * a3 * s + 12 * a4 * s^2 + 20 * a5 * s^3
    start_s2 = start_s * start_s;
    start_s3 = start_s2 * start_s;
    start_s4 = start_s3 * start_s;
    start_s5 = start_s4 * start_s;
    end_s2 = end_s * end_s;
    end_s3 = end_s2 * end_s;
    end_s4 = end_s3 * end_s;
    end_s5 = end_s4 * end_s;
    A = [1,start_s, start_s2,     start_s3,     start_s4,      start_s5;
         0 1,       2 * start_s,  3 * start_s2, 4 * start_s3,  5 * start_s4;
         0 0,       2,            6 * start_s,  12 * start_s2, 20 * start_s3;
         1,end_s, end_s2,     end_s3,     end_s4,      end_s5;
         0,1,     2 * end_s,  3 * end_s2, 4 * end_s3,  5 * end_s4;
         0,0,     2,          6 * end_s,  12 * end_s2, 20 * end_s3;];
    B = [start_l;
         start_dl;
         start_ddl;
         end_l;
         end_dl;
         end_ddl;];
     coeff = A \ B; 
end

== matlab function LATC_Test_Calc/LCS_Angle/Trajectory_Planning/MATLAB Function4 ==
  data: X input; y output; Y input
function y = fcn(X,Y)

y = zeros(length(X),9);
for i = 1:1:length(X)
    y(i,1) = X(i);
    y(i,2) = Y(i);
    y(i,3) = 0;
    y(i,4) = 0;
    y(i,5) = 1;
    y(i,6) = i;
    y(i,7) = 0;
    y(i,8) = 1;
end
end

== matlab function LATC_Test_Calc/LCS_Angle/Trajectory_Planning/DP_Path/MATLAB Function1 ==
  data: X input; y output; Y input
function y = fcn(X,Y)

y = zeros(length(X),9);
for i = 1:1:length(X)
    y(i,1) = X(i);
    y(i,2) = Y(i);
    y(i,3) = 0;
    y(i,4) = 0;
    y(i,5) = 1;
    y(i,6) = i;
    y(i,7) = 0;
    y(i,8) = 1;
end
end

== matlab function LATC_Test_Calc/LCS_Angle/Trajectory_Planning/QP_Path/path planning with quadratic programming (qp)1 ==
  data: kappa_max input; l_min input; qp_path_l output; l_max input; w_cost_l input; w_cost_dl input; w_cost_ddl input; w_cost_dddl input; w_cost_centre input; w_cost_end_l input; w_cost_end_dl input; w_cost_end_ddl input; host_d1 input; host_d2 input; host_w input; plan_start_l input; plan_start_dl input; plan_start_ddl input; qp_path_dl output; qp_path_ddl output; dp_path_l_final input
function [qp_path_l,qp_path_dl,qp_path_ddl] = ...
fcn(kappa_max,l_min,l_max,w_cost_l,w_cost_dl,w_cost_ddl,w_cost_dddl,w_cost_centre,w_cost_end_l,w_cost_end_dl,w_cost_end_ddl,...
    host_d1,host_d2,host_w,...
    plan_start_l,plan_start_dl,plan_start_ddl,dp_path_l_final)
% 路径二次规划
% 0.5*x'Hx + f'*x = min
% subject to A*x <= b
%            Aeq*x = beq
%            lb <= x <= ub;
% 输入：l_min l_max 点的凸空间
%       w_cost_l 参考线代价
%       w_cost_dl ddl dddl 光滑性代价
%       w_cost_centre 凸空间中央代价
%       w_cost_end_l dl dd1 终点的状态代价 (希望path的终点状态为(0,0,0))
%       host_d1,d2 host质心到前后轴的距离
%       host_w host的宽度
%       plan_start_l,dl,ddl 规划起点
% 输出 qp_path_l dl ddl 二次规划输出的曲线
% coder.extrinsic("quadprog");
% 待优化的变量的数量
n = single(60);
%输出初始化
qp_path_l = single(zeros(n,1));
qp_path_dl = single(zeros(n,1));
qp_path_ddl = single(zeros(n,1));
% 构建约束
% subject to A*x <= b
%            Aeq*x = beq
%            lb <= x <= ub;
% Aeq_sub = [1 ds ds^2/3 -1 0 ds^2/6;
%            0 1  ds/2   0 -1 ds/2];
% x = [Li Li' Li'' Li+1 Li+1' Li+1'']
% beq = [0;0]

%-------------------以下为约束生成----------------
% 等式约束
Aeq = single(zeros(2*n-2,3*n));
beq = single(zeros(2*n-2,1));
% 两点间距ds = 1
ds = single(1);
Aeq_sub = single([1 ds ds^2/3 -1 0 ds^2/6;
                  0 1  ds/2   0 -1 ds/2]);
% 通过Aeq_sub填充Aeq ,beq不变全为0
for i = 1:n-1
    row = 2*i-1;
    col = 3*i-2;  
    Aeq(row:row+1,col:col+5) = Aeq_sub;  
end
% 不等式约束 A*x <= b
% 车辆四个角点在凸空间内
% 不等式矩阵初始化
A = single(zeros(8*n, 3*n));
b = single(zeros(8*n, 1));
%构建A_sub
d1 = host_d1;%质心到前保险杠距离
d2 = host_d2;%质心到后保险杠距离
w = host_w;%车宽
A_sub = [1  d1 0;
         1  d1 0;
         1 -d2 0;
         1 -d2 0;
        -1 -d1 0;
        -1 -d1 0;
        -1  d2 0;
        -1  d2 0];
% 生成A矩阵
for i=1:n
    row = 8*i-7;
    col = 3*i-2;
    A(row:row+7,col:col+2) = A_sub;
end
% 这里没有对曲率做强制约束，并不好
% 可以用 |dl(i+1) - dl(i)|/ds <= kappa_max 近似去约束曲率
% 以下为对曲率进行约束
A_cur = single(zeros(n-1,3*n));
b_cur = single(ones(n-1,1)*kappa_max);
A_cur_sub = single([-1 0 0 1 0 0]);
for i = 1:n-1
    row = i;
    col = 3*i-2;
    A_cur(row,col:col+5) = A_cur_sub;
end


% 生成b矩阵
% 只要找到四个角点所对应的l_min l_max 即可
% 。。。。。。。。。。。。。。
%    [    .   ]<- 
%    [        ]
% 。。。。。。。。。。。。。
front_index = ceil(d1/ds);
back_index = ceil(d2/ds);
for i=1:n
    index1 = min(i+front_index,n);
    index2 = max(i-back_index,1);
    b(8*i - 7:8*i,1) = [l_max(index1) - w/2;
                        l_max(index1) + w/2;
                        l_max(index2) - w/2;
                        l_max(index2) + w/2;
                       -l_min(index1) + w/2;
                       -l_min(index1) - w/2;
                       -l_min(index2) + w/2;
                       -l_min(index2) - w/2;];
end
%生成边界约束lb ub。主要是对规划起点做约束
lb = single(ones(3*n,1)*-inf);
ub = single(ones(3*n,1)*inf);
lb(1) = plan_start_l;
lb(2) = plan_start_dl;
lb(3) = plan_start_ddl;
ub(1) = lb(1);
ub(2) = lb(2);
ub(3) = lb(3);
%------------------以上约束生成完毕--------------------------
%------------------生成H矩阵--------------------------------
% 矩阵初始化
H_L = zeros(3*n, 3*n);
H_DL = zeros(3*n, 3*n);
H_DDL = zeros(3*n, 3*n);
H_DDDL = zeros(n-1, 3*n);
H_CENTRE = zeros(3*n, 3*n);
H_L_END = zeros(3*n, 3*n);
H_DL_END = zeros(3*n, 3*n);
H_DDL_END = zeros(3*n, 3*n);
% 生成H_L,H_DL,H_DDL,H_CENTRE
for i = 1:n
    H_L(3*i - 2,3*i - 2) = 1;
    H_DL(3*i - 1,3*i - 1) = 1;
    H_DDL(3*i, 3*i) = 1;
end
H_CENTRE = H_L; %尽量沿着dp轨迹走
% 生成H_DDDL;
H_dddl_sub = [0 0 1 0 0 -1];
for i = 1:n-1
    row = i;
    col = 3*i - 2;
    H_DDDL(row,col:col + 5) = H_dddl_sub;
end
% 生成H_L_END H_DL_END H_DDL_END
H_L_END(3*n - 2,3*n - 2) = 1;
H_DL_END(3*n - 1,3*n - 1) = 1;
H_DDL_END(3*n,3*n) = 1;
% 生成二次规划的H
H = w_cost_l * (H_L'*H_L) + w_cost_dl * (H_DL'*H_DL) + w_cost_ddl * (H_DDL'*H_DDL)...
   +w_cost_dddl * (H_DDDL'*H_DDDL) + w_cost_centre * (H_CENTRE'*H_CENTRE) + w_cost_end_l * (H_L_END'*H_L_END)...
   +w_cost_end_dl * (H_DL_END'* H_DL_END) + w_cost_ddl * (H_DDL_END'*H_DDL_END);
H = single(2 * H);
%---------------------------生成H完毕------------------------------
% 0.5*x'Hx + f'*x = min
% 生成f
f = single(zeros(3*n,1));
%centre_line = 0.5 * (l_min + l_max);
centre_line = dp_path_l_final;
for i = 1:n
    f(3*i - 2) = -2 * centre_line(i);
end
f = w_cost_centre * f;
% 终点要接近end_l dl ddl desire
%  期望的终点状态
end_l_desire = 0;
end_dl_desire = 0;
end_ddl_desire = 0;
f(3*n - 2) = f(3*n - 2) -2 * end_l_desire * w_cost_end_l;
f(3*n - 1) = f(3*n - 1) -2 * end_dl_desire * w_cost_end_dl;
f(3*n) = f(3*n) -2 * end_ddl_desire * w_cost_end_ddl;
%-----------f构造完毕---------------------------------------------
% 0.5*x'Hx + f'*x = min
% subject to A*x <= b
%            Aeq*x = beq
%            lb <= x <= ub;

% X = quadprog(H,f,A,b,Aeq,beq,lb,ub);

%---------改造求解---------------
% J = 0.5x'Hx + f'x = min
% A_Const * x <= b
A_Const = single([A;eye(3*n,3*n);-1*eye(3*n,3*n);Aeq;-1*Aeq;A_cur;-1*A_cur]);
b_Const = single([b;ub;-1*lb;beq;-1*beq;b_cur;b_cur]);

X = MPC_Solver_QPhild(H,f,A_Const,b_Const);

for i = 1:n
    qp_path_l(i) = X(3*i - 2);
    qp_path_dl(i) = X(3*i - 1);
    qp_path_ddl(i) = X(3*i);
end

end
function eta = MPC_Solver_QPhild(H,f,A_Const,b)
% 二次规划
% 该算法是原始对偶算法，该方法充分的剖析了优化问题的结构，是求解二次规划问题的一个较好的算法。
% J = 0.5x'Hx + f'x = min
% A_Const*x <= b
[n1,~] = size(A_Const);
eta = -H\f;
kk = uint8(0);
for i = 1:n1
    if(A_Const(i,:)*eta>b(i))
        kk = kk+uint8(1);
    else
        kk = kk+uint8(0);
    end
end
if kk == uint8(0)
    return;
end
P = A_Const*(H\A_Const');
d = (A_Const*(H\f)+b);
[n,m] = size(d);
x_ini = zeros(n,m);
lambda = x_ini;
al = single(10);
for km = 1:38
    lambda_p = lambda;
    for i = 1:n
        w = P(i,:)*lambda - P(i,i)*lambda(i,1);
        w = w + d(i,1);
        la = -w/P(i,i);
        lambda(i,1) = max(0,la);
    end
    al = (lambda - lambda_p)'*(lambda - lambda_p);
    if(al<10e-8)
        break
    end
end
eta = -H\f -H\A_Const'*lambda;
end

== matlab function LATC_Test_Calc/LCS_Angle/Trajectory_Planning/DP_Path/MATLAB Function14 ==
  data: X input; y output; Y input
function y = fcn(X,Y)

y = zeros(length(X),9);
for i = 1:1:length(X)
    y(i,1) = X(i);
    y(i,2) = Y(i);
    y(i,3) = 0;
    y(i,4) = 0;
    y(i,5) = 1;
    y(i,6) = i;
    y(i,7) = 0;
    y(i,8) = 1;
end
end

== matlab function LATC_Test_Calc/LCS_Angle/Trajectory_Points/MATLAB Function1 ==
  data: CenterLinePointX input; CenterLinePoint2_X output single; CenterLinePointY input; CenterLinePoint2_Y output single
function [CenterLinePoint2_X,CenterLinePoint2_Y]= fcn(CenterLinePointX,CenterLinePointY)
CenterLinePoint = single(zeros(300,2));
CenterLinePoint2_X = single(zeros(100,1));
CenterLinePoint2_Y = single(zeros(100,1));

CenterLinePoint = [CenterLinePointX CenterLinePointY];

% MinDisPtX = single(zeros(1,1));
% MinDisPtY = single(zeros(1,1));
PtNum = single(length(CenterLinePoint));
Index = single(300);
MinDis = single(10000);
i = single(1);
while(i < PtNum)
    Dis = single(sqrt((0-CenterLinePointX(i,1))*(0-CenterLinePointX(i,1)) + (0-CenterLinePointY(i,1))*(0-CenterLinePointY(i,1))));
    if(Dis < MinDis)
        MinDis = Dis;
        Index = i;
    end
    i = i + 1;
end
% MinDisPtX(1,1) = CenterLinePointX(Index,1);
% MinDisPtY(1,1) = CenterLinePointY(Index,1);

% Star_Index = find((CenterLinePoint(:,1) >=0 & CenterLinePoint(:,1) <=2) & (abs(CenterLinePoint(:,2)) <= 5),1,'first')
% Star_Index = single(0);
% Star_Index = find((CenterLinePoint(:,1) == MinDisPtX & CenterLinePoint(:,2) == MinDisPtY))
Star_Index = Index;

if  (Star_Index + 100) > 300
    for i = 1:1:(301 - Star_Index)
        CenterLinePoint2_X(i,1) = CenterLinePointX(Star_Index+i-1,1);
        CenterLinePoint2_Y(i,1) = CenterLinePointY(Star_Index+i-1,1);
    end
    for i = (301 - Star_Index):1:100
        CenterLinePoint2_X(i,1) = CenterLinePointX(end,1);
        CenterLinePoint2_Y(i,1) = CenterLinePointY(end,1);
    end

else
    for i = 1:1:100
        Pt_Num = length(CenterLinePointX);
        Select_Index = (ceil(linspace(Star_Index,Pt_Num,100)))';
        CenterLinePoint2_X(i,1) = CenterLinePointX(Select_Index(i,1),1);
        CenterLinePoint2_Y(i,1) = CenterLinePointY(Select_Index(i,1),1);
    end
end

end

== matlab function LATC_Test_Calc/LCS_Angle/Trajectory_Planning/MATLAB Function2 ==
  data: Ref_X input; s output single; Ref_Y input; sDot output single; sDotDot output single; l output single; lPrime output single; lPrimePrime output single; VehSpd input
function [s, sDot, sDotDot, l, lPrime, lPrimePrime]= FrenetStateCalc(Ref_X,Ref_Y,VehSpd)
s=single(zeros(1,1));sDot=single(zeros(1,1)); sDotDot=single(zeros(1,1)); l=single(zeros(1,1)); lPrime=single(zeros(1,1)); lPrimePrime=single(zeros(1,1));
rx = single(-1.*Ref_Y);
ry = Ref_X;
waypoints = [rx,ry];
referencePathPointNum = 100; %参考轨迹的点的个数(参考点的分辨率)，此参数会影响最终目标轨迹线的形状，太小会出现轨迹线拐点
referencePath = FrenentReferencePath(waypoints,referencePathPointNum);
%% 定义轨迹起始点状态
initGlobalState = [0 0 pi/2 0 VehSpd  0]; %暂时定义纵向加速度为0，[x, y,theta, kappa speed，Acc]
initFrenetState = referencePath.global2frenet(initGlobalState);
s = single(initFrenetState(1,1));
sDot = single(initFrenetState(1,2)); 
sDotDot = single(initFrenetState(1,3)); 
l = single(initFrenetState(1,4));
lPrime = single(initFrenetState(1,5));
lPrimePrime = single(initFrenetState(1,6));
end

== matlab function LATC_Test_Calc/LCS_Angle/Trajectory_Points/RoadCreate1/MATLAB Function1 ==
  data: A0 input size=[1 1]; CenterLinePointX output; A1 input size=[1 1]; A2 input size=[1 1]; A3 input size=[1 1]; CenterLinePointY output
function [CenterLinePointX,CenterLinePointY]= LineDiscrete(A0,A1,A2,A3)
CenterLinePointX = single(zeros(300,1));
CenterLinePointY = single(zeros(300,1));
CenterLinePointX = (single(linspace(0,150,300)))';
CenterLinePointY = A0 + A1.*CenterLinePointX + A2.*CenterLinePointX.^2 + A3.*CenterLinePointX.^3;
end
